simulink subsystem "OriginalLoadEstimator"  (R2022a)
settings: Solver=VariableStepAuto  StartTime=0.0  StopTime=10.0  RelTol=1e-3
model mask{w=0, dMdTheta=0}
  mask prompts: w "bandwidth"
undefined symbols (not defined in the file): DT
settings Model: Creator=jhummel  LastModifiedBy=jhummel

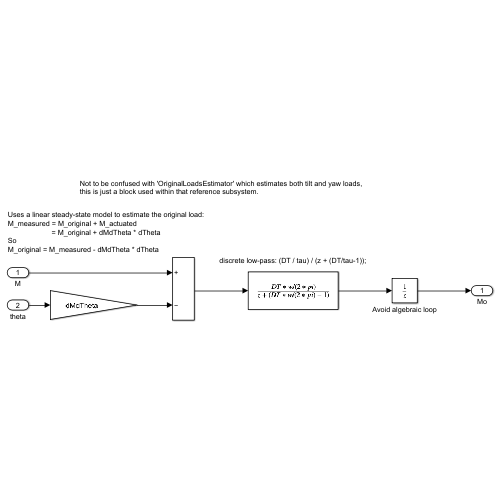
[thumbnail: Simulink's stored preview of the top-level diagram]
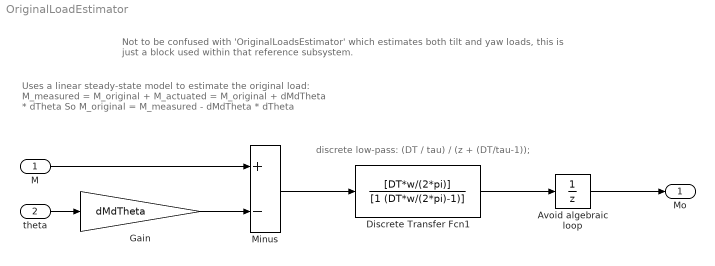
== system OriginalLoadEstimator ==
  note: Not to be confused with 'OriginalLoadsEstimator' which estimates both tilt and yaw loads, this is just a block used within that reference subsystem.
  note: Uses a linear steady-state model to estimate the original load:
      | M_measured = M_original + M_actuated
      |                       = M_original + dMdTheta * dTheta
      | So
      | M_original = M_measured - dMdTheta * dTheta
  note: discrete low-pass: (DT / tau) / (z + (DT/tau-1));
  M : Inport
  theta : Inport  Port=2
  Avoid algebraic loop : UnitDelay  SampleTime=-1  HasFrameUpgradeWarning=on
  Discrete Transfer Fcn1 : DiscreteTransferFcn  Numerator=[DT*w/(2*pi)]  Denominator=[1 (DT*w/(2*pi)-1)]
  Gain : Gain  Gain=dMdTheta
  Minus : Sum  Inputs=+-
  Mo : Outport
  wires:
  Minus/1 -> Discrete Transfer Fcn1/1
  theta/1 -> Gain/1
  M/1 -> Minus/1
  Avoid algebraic loop/1 -> Mo/1
  Discrete Transfer Fcn1/1 -> Avoid algebraic loop/1
  Gain/1 -> Minus/2
